simulink model "x4bus_model"  (R2024b)
settings: Solver=VariableStepAuto  StartTime=0.0  StopTime=4  RelTol=1e-3
InitFcn:
  |         %主电路参数
  | Vin = 800;    Vtri = 400;
  | Vg = 220;     Po = 100e3*1; Qo=0;
  | Po2 = Po;    Qo2 = 0;
  | Vg1 = Vg;
  | fline = 50;   fsw = 10e3;
  | fsample = 20e3;
  | wn = 2*pi*fline;
  | L1 = 3.2e-3;  C = 50e-6;
  | L2 = 800e-6;
  | Rcf = 0.8;
  | %% GFM1
  |         %有功功率环路参数
  | Dp = 1.59e4;  %EN 50438 要求频率变化49~51Hz
  | J = 0.081;
  |         %无功功率环路参数
  | Dq = 3210;
  | K = 7.1;
  | 
  | Rv = 0.6;Lv = 3.2e-3;
  | Kp_Vreg = 0.4;
  | Ki_Vreg = 90;
  | Kp_Ireg = 11;
  | Ki_Ireg = 0;
  | 
  | Ts = 1e-6;
  | 
  | t1 = 5;
  | t2 = 100;
  | 
  | %% GFM2
  |         %有功功率环路参数
  | Dp2 = 1.59e4;  %EN 50438 要求频率变化49~51Hz
  | J2 = 0.081;
  |         %无功功率环路参数
  | Dq2 = 3210;
  | K2 = 7.1;
  | 
  | Rv2 = 0.46;Lv2 = 0.8e-3;
  | Kp_Vreg2 = 0.3;   % 0.25
  | Ki_Vreg2 = 85;    % 80
  | Kp_Ireg2 = 11;
  | Ki_Ireg2 = 0;
undefined symbols (not defined in the file or in its folder): DiscIntNeverNeededParam, t_C, t_R
libraries: spsThreePhaseSeriesRLCBranchLib x13, spsCurrentMeasurementLib x12, spsControlledVoltageSourceLib x9, slpidlib x8, spsGroundLib x7, spsabctodq0Lib x6, spsVoltageMeasurementLib x6, spsThreePhaseBreakerLib x4, spsdq0toabcLib x3, spsFirstOrderFilterLib x2, sps_lib x1
(part 1 of 2)
settings Model: Creator=ZhenWei  LastModifiedBy=ZhenWei
settings DataIOCC: ReturnWorkspaceOutputs=off

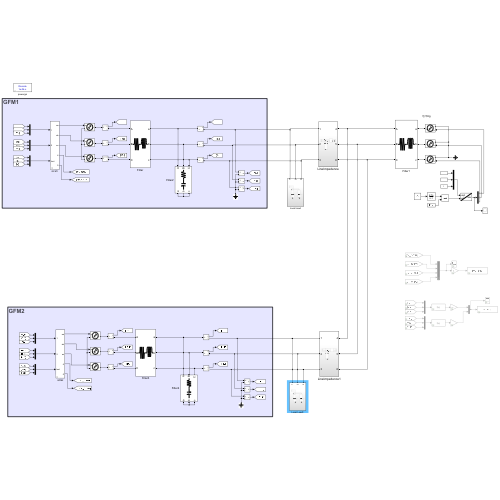
[thumbnail: Simulink's stored preview of the top-level diagram]
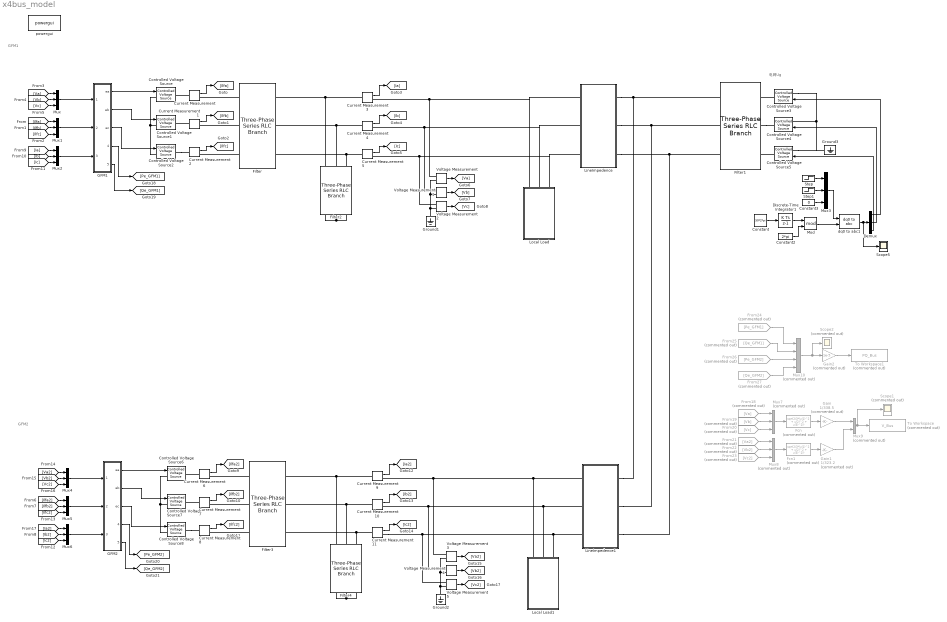
== system x4bus_model ==
  note: GFM1
  note: 电网Ug
  note: GFM2
  Constant : Constant  Value=50*2*pi
  Constant2 : Constant  Value=2*pi
  Constant3 : Constant  Value=0
  Controlled Voltage Source{,1..8} (9 alike) : spsControlledVoltageSourceLib/Controlled Voltage Source  Initialize=on  Source_Type=AC  Amplitude=0  Phase=0  Frequency=0  Measurements=None
  Current Measurement{,1..11} (12 alike) : spsCurrentMeasurementLib/Current Measurement  PhasorSimulation=off  OutputType=Complex  PSBequivalent=0
  Demux : Demux  Outputs=3
  Discrete-Time Integrator1 : DiscreteIntegrator  SampleTime=-1  ICPrevOutput=DiscIntNeverNeededParam  ICPrevScaledInput=DiscIntNeverNeededParam
  Fcn : Fcn  Commented=on  Expr=sqrt(2/3*(u(1)^2 + u(2)^2 + u(3)^2))
  Fcn1 : Fcn  Commented=on  Expr=sqrt(2/3*(u(1)^2 + u(2)^2 + u(3)^2))
  Filter : spsThreePhaseSeriesRLCBranchLib/Three-Phase Series RLC Branch  LConnTagsString=A|B|C  RConnTagsString=A|B|C  BranchType=RL  Resistance=0.05  Inductance=L1  Capacitance=1e-6  Measurements=None
  Filter1 : spsThreePhaseSeriesRLCBranchLib/Three-Phase Series RLC Branch  LConnTagsString=A|B|C  RConnTagsString=A|B|C  BranchType=RL  Resistance=0.01452  Inductance=0.462e-3  Capacitance=1e-6  Measurements=None
  Filter2 : spsThreePhaseSeriesRLCBranchLib/Three-Phase Series RLC Branch  LConnTagsString=A|B|C  RConnTagsString=A|B|C  BranchType=RC  Resistance=Rcf  Inductance=L2  Capacitance=C  Measurements=None
  Filter3 : spsThreePhaseSeriesRLCBranchLib/Three-Phase Series RLC Branch  LConnTagsString=A|B|C  RConnTagsString=A|B|C  BranchType=RL  Resistance=0.05  Inductance=L1  Capacitance=1e-6  Measurements=None
  Filter4 : spsThreePhaseSeriesRLCBranchLib/Three-Phase Series RLC Branch  LConnTagsString=A|B|C  RConnTagsString=A|B|C  BranchType=RC  Resistance=Rcf  Inductance=L2  Capacitance=C  Measurements=None
  From18 : From  Commented=on  GotoTag=Va
  From19 : From  Commented=on  GotoTag=Vb
  From20 : From  Commented=on  GotoTag=Vc
  From21 : From  Commented=on  GotoTag=Va2
  From22 : From  Commented=on  GotoTag=Vb2
  From23 : From  Commented=on  GotoTag=Vc2
  From24 : From  Commented=on  GotoTag=Pe_GFM1
  From25 : From  Commented=on  GotoTag=Qe_GFM1
  From26 : From  Commented=on  GotoTag=Pe_GFM2
  From27 : From  Commented=on  GotoTag=Qe_GFM2
  GFM1 : Subsystem  mask{J=J, Dp=Dp, Dq=Dq, K=K, Kp_Vreg=Kp_Vreg, Ki_Vreg=Ki_Vreg, Kp_Ireg=Kp_Ireg, Ki_Ireg=Ki_Ireg, Lv=Lv, Rv=Rv, Po=Po, Qo=Qo}
      mask prompts: J "惯性系数J"; Dp "有功阻尼Dp"; Dq "无功阻尼Dq"; K "下垂系数K"; Kp_Vreg "电压环kp"; Ki_Vreg "电压环ki"; Kp_Ireg "电流环kp"; Ki_Ireg "电流环ki"; Lv "虚拟电感Lv"; Rv "虚拟电阻Rv"; Po "有功功率Po"; Qo "无功功率Qo"
      mask DialogControl ParameterGroupVar Prompt: 参数
  GFM2 : Subsystem  mask{J=J2, Dp=Dp2, Dq=Dq2, K=K2, Kp_Vreg=Kp_Vreg2, Ki_Vreg=Ki_Vreg2, Kp_Ireg=Kp_Ireg2, Ki_Ireg=Ki_Ireg2, Lv=Lv2, Rv=Rv2, Po=Po2, Qo=Qo2}
      mask prompts: J "惯性系数J"; Dp "有功阻尼Dp"; Dq "无功阻尼Dq"; K "下垂系数K"; Kp_Vreg "电压环kp"; Ki_Vreg "电压环ki"; Kp_Ireg "电流环kp"; Ki_Ireg "电流环ki"; Lv "虚拟电感Lv"; Rv "虚拟电阻Rv"; Po "有功功率Po"; Qo "无功功率Qo"
      mask DialogControl ParameterGroupVar Prompt: 参数
  Gain : Gain  Commented=on  Gain=1/338.5
  Gain1 : Gain  Commented=on  Gain=1/323.2
  Gain2 : Gain  Commented=on  Gain=1e-5
  Ground1 : spsGroundLib/Ground  LConnTagsString=a
  Ground2 : spsGroundLib/Ground  LConnTagsString=a
  Ground3 : spsGroundLib/Ground  LConnTagsString=a
  LineImpedence : Subsystem
  LineImpedence1 : Subsystem
  Local Load : Subsystem
  Local Load1 : Subsystem
  Mod : Math  Operator=mod
  Mux{,1..6} (7 alike) : Mux  Inputs=3
  Mux10 : Mux  Commented=on
  Mux7 : Mux  Commented=on  Inputs=3
  Mux8 : Mux  Commented=on  Inputs=3
  Mux9 : Mux  Commented=on  Inputs=2
  Scope1 : Scope  Commented=on
  Scope2 : Scope  Commented=on
  Scope5 : Scope
  Step : Step  Time=10  Before=311  After=311+20  SampleTime=0
  Step1 : Step  Time=10  After=30  SampleTime=0
  To Workspace : ToWorkspace  Commented=on  VariableName=V_Bus  SaveFormat=Timeseries  SampleTime=-1
  To Workspace1 : ToWorkspace  Commented=on  VariableName=PQ_Bus  SaveFormat=Timeseries  SampleTime=-1
  Voltage Measurement{,1..5} (6 alike) : spsVoltageMeasurementLib/Voltage Measurement  PhasorSimulation=off  OutputType=Complex  PSBequivalent=0
  dq0 to abc1 : spsdq0toabcLib/dq0 to abc  Alignment=90 degrees behind phase A axis
  powergui : sps_lib/powergui  Priority=1  SimulationMode=Discrete  SampleTime=1e-6  frequency=60  Iterations=50  frequencyindice=0  Pbase=100e6  ErrMax=1e-4  UnitsV=kV  UnitsW=MW  buscounter=0  FunctionMessages=off  echomessages=off  EnableUseOfTLC=off  CurrentSourceSwitches=off  DisableSnubberDevices=off  DisableRonSwitches=off  DisableVfSwitches=off  DisplayEquations=off  AutomaticDiscreteSolvers=off  SolverType=Tustin/Backward Euler (TBE)  Interpol=off  ExternalGateDelay=off  methode=off  Ts=100  x0status=blocks  SPID=on  SwTol=0  HookPort=off  NonlinearTolerance=1e-4  nMaxIteration=100  ContinueOnMaxIteration=off  RestoreLinks=warning  ResistiveCurrentMeasurement=off  Frange=[0:2:500]  Ylog=off  Xlog=on  ShowGrid=off  save=off  variable=ZData  structure=0  ZoomFFT=off  StartTime=0.0  cycles=1  DisplayStyle=1  fundamental=60  FreqAxis=off  MaxFrequency=1000  frequencyindicesteady=1  RmsSteady=1  display=off
  wires:
  Current Measurement/1 -> [Ilfa]
  Current Measurement1/1 -> [Ilfb]
  Current Measurement2/1 -> [Ilfc]
  Current Measurement3/1 -> [Ia]
  Current Measurement4/1 -> [Ib]
  Current Measurement5/1 -> [Ic]
  Voltage Measurement/1 -> [Va]
  Voltage Measurement1/1 -> [Vb]
  Voltage Measurement2/1 -> [Vc]
  GFM1/1(ea) -> Controlled Voltage Source/1
  GFM1/2(eb) -> Controlled Voltage Source1/1
  GFM1/3(ec) -> Controlled Voltage Source2/1
  [Va] -> Mux/1
  [Vb] -> Mux/2
  [Vc] -> Mux/3
  [Ilfa] -> Mux1/1
  [Ilfb] -> Mux1/2
  [Ilfc] -> Mux1/3
  [Ic] -> Mux2/3
  [Ib] -> Mux2/2
  [Ia] -> Mux2/1
  Mux/1 -> GFM1/1(Inport)
  Mux1/1 -> GFM1/2(Inport1)
  Mux2/1 -> GFM1/3(Iout)
  Constant/1 -> Discrete-Time Integrator1/1
  Discrete-Time Integrator1/1 -> Mod/1
  Constant2/1 -> Mod/2
  Mod/1 -> dq0 to abc1/2
  Step/1 -> Mux3/1
  Constant3/1 -> Mux3/3
  Mux3/1 -> dq0 to abc1/1
  dq0 to abc1/1 -> Scope5/1, Demux/1
  Demux/1 -> Controlled Voltage Source3/1
  Demux/2 -> Controlled Voltage Source4/1
  Demux/3 -> Controlled Voltage Source5/1
  Step1/1 -> Mux3/2
  Mux6/1 -> GFM2/3(Iout)
  Mux5/1 -> GFM2/2(Inport1)
  Mux4/1 -> GFM2/1(Inport)
  [Ia2] -> Mux6/1
  [Ib2] -> Mux6/2
  [Ic2] -> Mux6/3
  [Ilfc2] -> Mux5/3
  [Ilfb2] -> Mux5/2
  [Ilfa2] -> Mux5/1
  [Vc2] -> Mux4/3
  [Vb2] -> Mux4/2
  [Va2] -> Mux4/1
  GFM2/3(ec) -> Controlled Voltage Source8/1
  GFM2/2(eb) -> Controlled Voltage Source7/1
  GFM2/1(ea) -> Controlled Voltage Source6/1
  Voltage Measurement5/1 -> [Vc2]
  Voltage Measurement4/1 -> [Vb2]
  Voltage Measurement3/1 -> [Va2]
  Current Measurement11/1 -> [Ic2]
  Current Measurement10/1 -> [Ib2]
  Current Measurement9/1 -> [Ia2]
  Current Measurement8/1 -> [Ilfc2]
  Current Measurement7/1 -> [Ilfb2]
  Current Measurement6/1 -> [Ilfa2]
  Mux7/1 -> Fcn/1
  From18/1 -> Mux7/1
  From19/1 -> Mux7/2
  From20/1 -> Mux7/3
  Fcn/1 -> Gain/1
  From23/1 -> Mux8/3
  From22/1 -> Mux8/2
  From21/1 -> Mux8/1
  Mux8/1 -> Fcn1/1
  Fcn1/1 -> Gain1/1
  Gain/1 -> Mux9/1
  Gain1/1 -> Mux9/2
  Mux9/1 -> Scope1/1, To Workspace/1
  GFM1/4(Out1) -> [Pe_GFM1]
  GFM1/5(Out2) -> [Qe_GFM1]
  GFM2/4(Out1) -> [Pe_GFM2]
  GFM2/5(Out2) -> [Qe_GFM2]
  Mux10/1 -> Scope2/1, Gain2/1
  From24/1 -> Mux10/1
  From25/1 -> Mux10/2
  From26/1 -> Mux10/3
  From27/1 -> Mux10/4
  Gain2/1 -> To Workspace1/1
  connections:
  Controlled Voltage Source/LConn1 -- Controlled Voltage Source2/LConn1 -- Controlled Voltage Source1/LConn1
  Current Measurement/LConn1 -- Controlled Voltage Source/RConn1
  Current Measurement1/LConn1 -- Controlled Voltage Source1/RConn1
  Controlled Voltage Source2/RConn1 -- Current Measurement2/LConn1
  Filter2/LConn2 -- Current Measurement4/LConn1 -- Filter/RConn2
  Filter2/LConn1 -- Current Measurement3/LConn1 -- Filter/RConn1
  Filter2/RConn1 -- Filter2/RConn2 -- Filter2/RConn3
  Filter2/LConn3 -- Current Measurement5/LConn1 -- Filter/RConn3
  Filter/LConn2 -- Current Measurement1/RConn1
  Filter/LConn1 -- Current Measurement/RConn1
  Filter/LConn3 -- Current Measurement2/RConn1
  Filter1/RConn2 -- Controlled Voltage Source4/RConn1
  Controlled Voltage Source3/RConn1 -- Filter1/RConn1
  Controlled Voltage Source5/RConn1 -- Filter1/RConn3
  Voltage Measurement/LConn1 -- LineImpedence/LConn1 -- Local Load/LConn1 -- Current Measurement3/RConn1
  Voltage Measurement1/LConn1 -- LineImpedence/LConn2 -- Local Load/LConn2 -- Current Measurement4/RConn1
  Voltage Measurement/LConn2 -- Voltage Measurement1/LConn2 -- Ground1/LConn1 -- Voltage Measurement2/LConn2
  Controlled Voltage Source3/LConn1 -- Controlled Voltage Source5/LConn1 -- Ground3/LConn1 -- Controlled Voltage Source4/LConn1
  Voltage Measurement2/LConn1 -- LineImpedence/LConn3 -- Local Load/LConn3 -- Current Measurement5/RConn1
  Controlled Voltage Source6/LConn1 -- Controlled Voltage Source7/LConn1 -- Controlled Voltage Source8/LConn1
  Filter4/LConn2 -- Current Measurement10/LConn1 -- Filter3/RConn2
  Filter4/LConn1 -- Current Measurement9/LConn1 -- Filter3/RConn1
  Filter4/RConn1 -- Filter4/RConn3 -- Filter4/RConn2
  Filter4/LConn3 -- Filter3/RConn3 -- Current Measurement11/LConn1
  Voltage Measurement3/LConn2 -- Voltage Measurement5/LConn2 -- Ground2/LConn1 -- Voltage Measurement4/LConn2
  Filter3/LConn3 -- Current Measurement8/RConn1
  Filter3/LConn2 -- Current Measurement7/RConn1
  Filter3/LConn1 -- Current Measurement6/RConn1
  Current Measurement7/LConn1 -- Controlled Voltage Source7/RConn1
  Controlled Voltage Source8/RConn1 -- Current Measurement8/LConn1
  Current Measurement6/LConn1 -- Controlled Voltage Source6/RConn1
  LineImpedence/RConn1 -- LineImpedence1/RConn1 -- Filter1/LConn1
  LineImpedence/RConn2 -- LineImpedence1/RConn2 -- Filter1/LConn2
  LineImpedence/RConn3 -- LineImpedence1/RConn3 -- Filter1/LConn3
  LineImpedence1/LConn1 -- Current Measurement9/RConn1 -- Voltage Measurement3/LConn1 -- Local Load1/LConn1
  LineImpedence1/LConn2 -- Local Load1/LConn2 -- Voltage Measurement4/LConn1 -- Current Measurement10/RConn1
  Current Measurement11/RConn1 -- Voltage Measurement5/LConn1 -- Local Load1/LConn3 -- LineImpedence1/LConn3

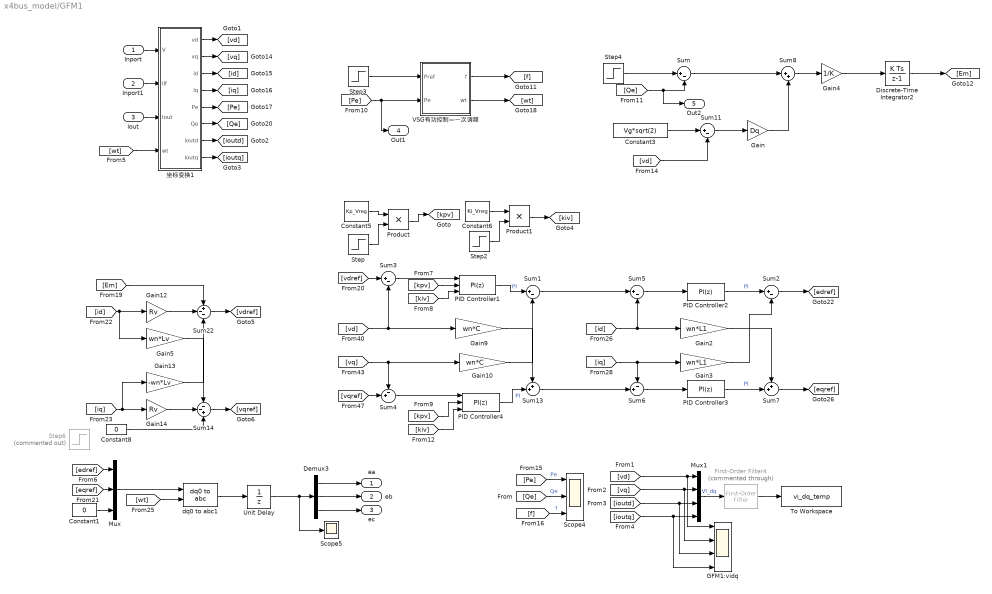
== system x4bus_model/GFM1 ==
  Inport : Inport
  Inport1 : Inport  Port=2
  Iout : Inport  Port=3
  Constant1 : Constant  Value=0
  Constant3 : Constant  Value=Vg*sqrt(2)
  Constant5 : Constant  Value=Kp_Vreg
  Constant6 : Constant  Value=Ki_Vreg
  Constant8 : Constant  Value=0
  Demux3 : Demux  Outputs=3
  Discrete-Time Integrator2 : DiscreteIntegrator  SampleTime=-1  ICPrevOutput=DiscIntNeverNeededParam  ICPrevScaledInput=DiscIntNeverNeededParam
  First-Order Filter4 : spsFirstOrderFilterLib/First-Order Filter  Commented=through  FilterType=Lowpass  Tc=5e-3  Ts=Ts  Initialize=off  Vac_Init=[0, 0, 1000]  Vdc_Init=0  PlotResponse=off  FreqRange="[0,  200,  1]"
  GFM1:vidq : Scope  NumInputPorts=4
  Gain : Gain  Gain=Dq
  Gain10 : Gain  Gain=wn*C
  Gain12 : Gain  Gain=Rv
  Gain13 : Gain  Gain=-wn*Lv
  Gain14 : Gain  Gain=Rv
  Gain2 : Gain  Gain=wn*L1
  Gain3 : Gain  Gain=wn*L1
  Gain4 : Gain  Gain=1/K
  Gain5 : Gain  Gain=wn*Lv
  Gain9 : Gain  Gain=wn*C
  Mux : Mux  Inputs=3
  Mux1 : Mux
  PID Controller1 : slpidlib/PID Controller  Controller=PI  Form=Parallel  TimeDomain=Discrete-time  UseExternalTs=off  SampleTime=-1  IntegratorMethod=Forward Euler  FilterMethod=Forward Euler  ControllerParametersSource=external  P=Kp_Vreg  I=Ki_Vreg  UseKiTs=off  D=0  UseExternalDerivativeSource=off  N=100  UseFilter=on  TunerSelectOption=Transfer Function Based (PID Tuner App)  InitialConditionSource=internal  InitialConditionForIntegrator=0  InitialConditionForFilter=0  DifferentiatorICPrevScaledInput=0  ExternalReset=none  TrackingMode=off  Kt=1  LimitOutput=off  SatLimitsSource=internal  UpperSaturationLimit=inf  LowerSaturationLimit=-inf  LinearizeAsGain=on  AntiWindupMode=none  Kb=1  LimitIntegrator=off  UpperIntegratorSaturationLimit=inf  LowerIntegratorSaturationLimit=-inf  POutMin=[]  POutMax=[]  IOutMin=[]  IOutMax=[]  DOutMin=[]  DOutMax=[]  NOutMin=[]  NOutMax=[]  SumOutMin=[]  SumOutMax=[]  SaturationOutMin=[]  SaturationOutMax=[]  PParamMin=[]  PParamMax=[]  IParamMin=[]  IParamMax=[]  DParamMin=[]  DParamMax=[]  NParamMin=[]  NParamMax=[]  KbParamMin=[]  KbParamMax=[]  KtParamMin=[]  KtParamMax=[]  KbOutMin=[]  KbOutMax=[]  KtOutMin=[]  KtOutMax=[]  IntegratorOutMin=[]  IntegratorOutMax=[]  FilterOutMin=[]  FilterOutMax=[]  SumI1OutMin=[]  SumI1OutMax=[]  SumI2OutMin=[]  SumI2OutMax=[]  SumI3OutMin=[]  SumI3OutMax=[]  SumI4OutMin=[]  SumI4OutMax=[]  SumDOutMin=[]  SumDOutMax=[]  DifferentiatorOutMin=[]  DifferentiatorOutMax=[]  FilterDiffOutCoefMin=[]  FilterDiffOutCoefMax=[]  ReciprocalOutMin=[]  ReciprocalOutMax=[]  SumDenOutMin=[]  SumDenOutMax=[]  SumNumOutMin=[]  SumNumOutMax=[]  DivideOutMin=[]  DivideOutMax=[]  UdiffTsProdOutMin=[]  UdiffTsProdOutMax=[]  NTsProdOutMin=[]  NTsProdOutMax=[]  UintegralTsProdOutMin=[]  UintegralTsProdOutMax=[]  UngainTsProdOutMin=[]  UngainTsProdOutMax=[]  ClampingZeroOutDataTypeStr=Inherit: Inherit via back propagation  ClampingZeroOutMin=[]  ClampingZeroOutMax=[]  FilterDenConstantOutDataTypeStr=Inherit: Inherit via back propagation  FilterDenConstantOutMin=[]  FilterDenConstantOutMax=[]  PCopyOutDataTypeStr=Inherit: Inherit via back propagation  PCopyOutMin=[]  PCopyOutMax=[]  NCopyOutDataTypeStr=Inherit: Inherit via back propagation  NCopyOutMin=[]  NCopyOutMax=[]  IntegratorContinuousStateAttributes=''  IntegratorStateMustResolveToSignalObject=off  IntegratorRTWStateStorageClass=Auto  FilterContinuousStateAttributes=''  FilterStateMustResolveToSignalObject=off  FilterRTWStateStorageClass=Auto  ParallelPVariant=ExternalParameters  IdealPVariant=Disabled  IVariant=ExternalParameters  DVariant=Disabled  IntegratorVariant=Discrete  SatVariant=Disabled  AWVariant=Passthrough  PCopyVariant=Disabled  TRVariant=Disabled  FdbkBlocksVariant=Forward  IdealPFdbkVariant=Disabled  SatFdbkVariant=Disabled  DerivativeFilterVariant=Disabled  NVariant=Disabled  NCopyVariant=Disabled_SignalSpec  FilterICVariant=Disabled  IntegratorICVariant=InternalICs  ExternalResetVariant=Disabled  TRSumVariant=Passthrough  SumFdbkVariant=Disabled  SumVariant=Sum_PI  TsampFilterVariant=InternalTs  TsampNgainVariant=Passthrough  TsampIntegralVariant=Disabled_SignalSpec  ExternalSaturationOutDataTypeStr=Inherit: Same as second input  DerivativeSourceVariant=Disabled  PreIntVariant=InternalPreInt
  PID Controller2 : slpidlib/PID Controller  Controller=PI  Form=Parallel  TimeDomain=Discrete-time  UseExternalTs=off  SampleTime=-1  IntegratorMethod=Forward Euler  FilterMethod=Forward Euler  ControllerParametersSource=internal  P=Kp_Ireg  I=Ki_Ireg  UseKiTs=off  D=0  UseExternalDerivativeSource=off  N=100  UseFilter=on  TunerSelectOption=Transfer Function Based (PID Tuner App)  InitialConditionSource=internal  InitialConditionForIntegrator=0  InitialConditionForFilter=0  DifferentiatorICPrevScaledInput=0  ExternalReset=none  TrackingMode=off  Kt=1  LimitOutput=off  SatLimitsSource=internal  UpperSaturationLimit=inf  LowerSaturationLimit=-inf  LinearizeAsGain=on  AntiWindupMode=none  Kb=1  LimitIntegrator=off  UpperIntegratorSaturationLimit=inf  LowerIntegratorSaturationLimit=-inf  POutMin=[]  POutMax=[]  IOutMin=[]  IOutMax=[]  DOutMin=[]  DOutMax=[]  NOutMin=[]  NOutMax=[]  SumOutMin=[]  SumOutMax=[]  SaturationOutMin=[]  SaturationOutMax=[]  PParamMin=[]  PParamMax=[]  IParamMin=[]  IParamMax=[]  DParamMin=[]  DParamMax=[]  NParamMin=[]  NParamMax=[]  KbParamMin=[]  KbParamMax=[]  KtParamMin=[]  KtParamMax=[]  KbOutMin=[]  KbOutMax=[]  KtOutMin=[]  KtOutMax=[]  IntegratorOutMin=[]  IntegratorOutMax=[]  FilterOutMin=[]  FilterOutMax=[]  SumI1OutMin=[]  SumI1OutMax=[]  SumI2OutMin=[]  SumI2OutMax=[]  SumI3OutMin=[]  SumI3OutMax=[]  SumI4OutMin=[]  SumI4OutMax=[]  SumDOutMin=[]  SumDOutMax=[]  DifferentiatorOutMin=[]  DifferentiatorOutMax=[]  FilterDiffOutCoefMin=[]  FilterDiffOutCoefMax=[]  ReciprocalOutMin=[]  ReciprocalOutMax=[]  SumDenOutMin=[]  SumDenOutMax=[]  SumNumOutMin=[]  SumNumOutMax=[]  DivideOutMin=[]  DivideOutMax=[]  UdiffTsProdOutMin=[]  UdiffTsProdOutMax=[]  NTsProdOutMin=[]  NTsProdOutMax=[]  UintegralTsProdOutMin=[]  UintegralTsProdOutMax=[]  UngainTsProdOutMin=[]  UngainTsProdOutMax=[]  ClampingZeroOutDataTypeStr=Inherit: Inherit via back propagation  ClampingZeroOutMin=[]  ClampingZeroOutMax=[]  FilterDenConstantOutDataTypeStr=Inherit: Inherit via back propagation  FilterDenConstantOutMin=[]  FilterDenConstantOutMax=[]  PCopyOutDataTypeStr=Inherit: Inherit via back propagation  PCopyOutMin=[]  PCopyOutMax=[]  NCopyOutDataTypeStr=Inherit: Inherit via back propagation  NCopyOutMin=[]  NCopyOutMax=[]  IntegratorContinuousStateAttributes=''  IntegratorStateMustResolveToSignalObject=off  IntegratorRTWStateStorageClass=Auto  FilterContinuousStateAttributes=''  FilterStateMustResolveToSignalObject=off  FilterRTWStateStorageClass=Auto  ParallelPVariant=InternalParameters  IdealPVariant=Disabled  IVariant=InternalParameters  DVariant=Disabled  IntegratorVariant=Discrete  SatVariant=Disabled  AWVariant=Passthrough  PCopyVariant=Disabled  TRVariant=Disabled  FdbkBlocksVariant=Forward  IdealPFdbkVariant=Disabled  SatFdbkVariant=Disabled  DerivativeFilterVariant=Disabled  NVariant=Disabled  NCopyVariant=Disabled_SignalSpec  FilterICVariant=Disabled  IntegratorICVariant=InternalICs  ExternalResetVariant=Disabled  TRSumVariant=Passthrough  SumFdbkVariant=Disabled  SumVariant=Sum_PI  TsampFilterVariant=InternalTs  TsampNgainVariant=Passthrough  TsampIntegralVariant=Disabled_SignalSpec  ExternalSaturationOutDataTypeStr=Inherit: Same as second input  DerivativeSourceVariant=Disabled  PreIntVariant=InternalPreInt
  PID Controller3 : slpidlib/PID Controller  Controller=PI  Form=Parallel  TimeDomain=Discrete-time  UseExternalTs=off  SampleTime=-1  IntegratorMethod=Forward Euler  FilterMethod=Forward Euler  ControllerParametersSource=internal  P=Kp_Ireg  I=Ki_Ireg  UseKiTs=off  D=0  UseExternalDerivativeSource=off  N=100  UseFilter=on  TunerSelectOption=Transfer Function Based (PID Tuner App)  InitialConditionSource=internal  InitialConditionForIntegrator=0  InitialConditionForFilter=0  DifferentiatorICPrevScaledInput=0  ExternalReset=none  TrackingMode=off  Kt=1  LimitOutput=off  SatLimitsSource=internal  UpperSaturationLimit=inf  LowerSaturationLimit=-inf  LinearizeAsGain=on  AntiWindupMode=none  Kb=1  LimitIntegrator=off  UpperIntegratorSaturationLimit=inf  LowerIntegratorSaturationLimit=-inf  POutMin=[]  POutMax=[]  IOutMin=[]  IOutMax=[]  DOutMin=[]  DOutMax=[]  NOutMin=[]  NOutMax=[]  SumOutMin=[]  SumOutMax=[]  SaturationOutMin=[]  SaturationOutMax=[]  PParamMin=[]  PParamMax=[]  IParamMin=[]  IParamMax=[]  DParamMin=[]  DParamMax=[]  NParamMin=[]  NParamMax=[]  KbParamMin=[]  KbParamMax=[]  KtParamMin=[]  KtParamMax=[]  KbOutMin=[]  KbOutMax=[]  KtOutMin=[]  KtOutMax=[]  IntegratorOutMin=[]  IntegratorOutMax=[]  FilterOutMin=[]  FilterOutMax=[]  SumI1OutMin=[]  SumI1OutMax=[]  SumI2OutMin=[]  SumI2OutMax=[]  SumI3OutMin=[]  SumI3OutMax=[]  SumI4OutMin=[]  SumI4OutMax=[]  SumDOutMin=[]  SumDOutMax=[]  DifferentiatorOutMin=[]  DifferentiatorOutMax=[]  FilterDiffOutCoefMin=[]  FilterDiffOutCoefMax=[]  ReciprocalOutMin=[]  ReciprocalOutMax=[]  SumDenOutMin=[]  SumDenOutMax=[]  SumNumOutMin=[]  SumNumOutMax=[]  DivideOutMin=[]  DivideOutMax=[]  UdiffTsProdOutMin=[]  UdiffTsProdOutMax=[]  NTsProdOutMin=[]  NTsProdOutMax=[]  UintegralTsProdOutMin=[]  UintegralTsProdOutMax=[]  UngainTsProdOutMin=[]  UngainTsProdOutMax=[]  ClampingZeroOutDataTypeStr=Inherit: Inherit via back propagation  ClampingZeroOutMin=[]  ClampingZeroOutMax=[]  FilterDenConstantOutDataTypeStr=Inherit: Inherit via back propagation  FilterDenConstantOutMin=[]  FilterDenConstantOutMax=[]  PCopyOutDataTypeStr=Inherit: Inherit via back propagation  PCopyOutMin=[]  PCopyOutMax=[]  NCopyOutDataTypeStr=Inherit: Inherit via back propagation  NCopyOutMin=[]  NCopyOutMax=[]  IntegratorContinuousStateAttributes=''  IntegratorStateMustResolveToSignalObject=off  IntegratorRTWStateStorageClass=Auto  FilterContinuousStateAttributes=''  FilterStateMustResolveToSignalObject=off  FilterRTWStateStorageClass=Auto  ParallelPVariant=InternalParameters  IdealPVariant=Disabled  IVariant=InternalParameters  DVariant=Disabled  IntegratorVariant=Discrete  SatVariant=Disabled  AWVariant=Passthrough  PCopyVariant=Disabled  TRVariant=Disabled  FdbkBlocksVariant=Forward  IdealPFdbkVariant=Disabled  SatFdbkVariant=Disabled  DerivativeFilterVariant=Disabled  NVariant=Disabled  NCopyVariant=Disabled_SignalSpec  FilterICVariant=Disabled  IntegratorICVariant=InternalICs  ExternalResetVariant=Disabled  TRSumVariant=Passthrough  SumFdbkVariant=Disabled  SumVariant=Sum_PI  TsampFilterVariant=InternalTs  TsampNgainVariant=Passthrough  TsampIntegralVariant=Disabled_SignalSpec  ExternalSaturationOutDataTypeStr=Inherit: Same as second input  DerivativeSourceVariant=Disabled  PreIntVariant=InternalPreInt
  PID Controller4 : slpidlib/PID Controller  Controller=PI  Form=Parallel  TimeDomain=Discrete-time  UseExternalTs=off  SampleTime=-1  IntegratorMethod=Forward Euler  FilterMethod=Forward Euler  ControllerParametersSource=external  P=Kp_Vreg  I=Ki_Vreg  UseKiTs=off  D=0  UseExternalDerivativeSource=off  N=100  UseFilter=on  TunerSelectOption=Transfer Function Based (PID Tuner App)  InitialConditionSource=internal  InitialConditionForIntegrator=0  InitialConditionForFilter=0  DifferentiatorICPrevScaledInput=0  ExternalReset=none  TrackingMode=off  Kt=1  LimitOutput=off  SatLimitsSource=internal  UpperSaturationLimit=inf  LowerSaturationLimit=-inf  LinearizeAsGain=on  AntiWindupMode=none  Kb=1  LimitIntegrator=off  UpperIntegratorSaturationLimit=inf  LowerIntegratorSaturationLimit=-inf  POutMin=[]  POutMax=[]  IOutMin=[]  IOutMax=[]  DOutMin=[]  DOutMax=[]  NOutMin=[]  NOutMax=[]  SumOutMin=[]  SumOutMax=[]  SaturationOutMin=[]  SaturationOutMax=[]  PParamMin=[]  PParamMax=[]  IParamMin=[]  IParamMax=[]  DParamMin=[]  DParamMax=[]  NParamMin=[]  NParamMax=[]  KbParamMin=[]  KbParamMax=[]  KtParamMin=[]  KtParamMax=[]  KbOutMin=[]  KbOutMax=[]  KtOutMin=[]  KtOutMax=[]  IntegratorOutMin=[]  IntegratorOutMax=[]  FilterOutMin=[]  FilterOutMax=[]  SumI1OutMin=[]  SumI1OutMax=[]  SumI2OutMin=[]  SumI2OutMax=[]  SumI3OutMin=[]  SumI3OutMax=[]  SumI4OutMin=[]  SumI4OutMax=[]  SumDOutMin=[]  SumDOutMax=[]  DifferentiatorOutMin=[]  DifferentiatorOutMax=[]  FilterDiffOutCoefMin=[]  FilterDiffOutCoefMax=[]  ReciprocalOutMin=[]  ReciprocalOutMax=[]  SumDenOutMin=[]  SumDenOutMax=[]  SumNumOutMin=[]  SumNumOutMax=[]  DivideOutMin=[]  DivideOutMax=[]  UdiffTsProdOutMin=[]  UdiffTsProdOutMax=[]  NTsProdOutMin=[]  NTsProdOutMax=[]  UintegralTsProdOutMin=[]  UintegralTsProdOutMax=[]  UngainTsProdOutMin=[]  UngainTsProdOutMax=[]  ClampingZeroOutDataTypeStr=Inherit: Inherit via back propagation  ClampingZeroOutMin=[]  ClampingZeroOutMax=[]  FilterDenConstantOutDataTypeStr=Inherit: Inherit via back propagation  FilterDenConstantOutMin=[]  FilterDenConstantOutMax=[]  PCopyOutDataTypeStr=Inherit: Inherit via back propagation  PCopyOutMin=[]  PCopyOutMax=[]  NCopyOutDataTypeStr=Inherit: Inherit via back propagation  NCopyOutMin=[]  NCopyOutMax=[]  IntegratorContinuousStateAttributes=''  IntegratorStateMustResolveToSignalObject=off  IntegratorRTWStateStorageClass=Auto  FilterContinuousStateAttributes=''  FilterStateMustResolveToSignalObject=off  FilterRTWStateStorageClass=Auto  ParallelPVariant=ExternalParameters  IdealPVariant=Disabled  IVariant=ExternalParameters  DVariant=Disabled  IntegratorVariant=Discrete  SatVariant=Disabled  AWVariant=Passthrough  PCopyVariant=Disabled  TRVariant=Disabled  FdbkBlocksVariant=Forward  IdealPFdbkVariant=Disabled  SatFdbkVariant=Disabled  DerivativeFilterVariant=Disabled  NVariant=Disabled  NCopyVariant=Disabled_SignalSpec  FilterICVariant=Disabled  IntegratorICVariant=InternalICs  ExternalResetVariant=Disabled  TRSumVariant=Passthrough  SumFdbkVariant=Disabled  SumVariant=Sum_PI  TsampFilterVariant=InternalTs  TsampNgainVariant=Passthrough  TsampIntegralVariant=Disabled_SignalSpec  ExternalSaturationOutDataTypeStr=Inherit: Same as second input  DerivativeSourceVariant=Disabled  PreIntVariant=InternalPreInt
  Product : Product
  Product1 : Product
  Scope4 : Scope  NumInputPorts=3
  Scope5 : Scope
  Step : Step  Time=t1  Before=1  After=0.85  SampleTime=0
  Step2 : Step  Time=t1  Before=1  After=0.9  SampleTime=0
  Step3 : Step  Time=t1  Before=Po  After=-1*Po  SampleTime=0
  Step4 : Step  Time=t1  Before=Qo  After=1*Po  SampleTime=0
  Step6 : Step  Commented=on  Time=10  After=20  SampleTime=0
  Sum{,1..3,5,11} (6 alike) : Sum  Inputs=|+-
  Sum13 : Sum  Inputs=++|
  Sum14 : Sum  Inputs=--+
  Sum22 : Sum  Inputs=+--
  Sum4 : Sum  Inputs=-+|
  Sum6 : Sum  Inputs=-+|
  Sum7 : Sum  Inputs=++|
  Sum8 : Sum  Inputs=|++
  To Workspace : ToWorkspace  VariableName=vi_dq_temp  SaveFormat=Timeseries  SampleTime=-1
  Unit Delay : UnitDelay  SampleTime=-1  HasFrameUpgradeWarning=on
  VSG有功控制—一次调频 : Subsystem
  dq0 to abc1 : spsdq0toabcLib/dq0 to abc  Alignment=90 degrees behind phase A axis
  坐标变换1 : Subsystem
  ea : Outport
  eb : Outport  Port=2
  ec : Outport  Port=3
  Out1 : Outport  Port=4
  Out2 : Outport  Port=5
  wires:
  [Pe] -> Scope4/1  "Pe"
  [f] -> Scope4/3  "f"
  [Qe] -> Scope4/2  "Qe"
  [vq] -> GFM1:vidq/2, Mux1/2
  [ioutd] -> GFM1:vidq/3, Mux1/3
  [vd] -> GFM1:vidq/1, Mux1/1
  [ioutq] -> GFM1:vidq/4, Mux1/4
  Mux1/1 -> First-Order Filter4/1  "VI_dq"
  First-Order Filter4/1 -> To Workspace/1
  Inport1/1 -> 坐标变换1/2(Ilf)
  [wt] -> 坐标变换1/4(wt)
  坐标变换1/1(vd) -> [vd]
  坐标变换1/2(vq) -> [vq]
  坐标变换1/3(id) -> [id]
  坐标变换1/4(iq) -> [iq]
  坐标变换1/5(Pe) -> [Pe]
  坐标变换1/6(Qe) -> [Qe]
  [wt] -> dq0 to abc1/2
  [edref] -> Mux/1
  [eqref] -> Mux/2
  Mux/1 -> dq0 to abc1/1
  Constant1/1 -> Mux/3
  dq0 to abc1/1 -> Unit Delay/1
  Demux3/1 -> ea/1
  Demux3/2 -> eb/1
  Demux3/3 -> ec/1
  Unit Delay/1 -> Scope5/1, Demux3/1
  Inport/1 -> 坐标变换1/1(V)
  坐标变换1/8(ioutq) -> [ioutq]
  坐标变换1/7(ioutd) -> [ioutd]
  Iout/1 -> 坐标变换1/3(Iout)
  Gain14/1 -> Sum14/2
  Gain12/1 -> Sum22/2
  [Em] -> Sum22/1
  Constant8/1 -> Sum14/3
  Sum14/1 -> [vqref]
  [id] -> Gain5/1, Gain12/1
  Gain13/1 -> Sum22/3
  Gain5/1 -> Sum14/1
  Sum22/1 -> [vdref]
  [iq] -> Gain13/1, Gain14/1
  [Pe] -> Out1/1, VSG有功控制—一次调频/2(Pe)
  VSG有功控制—一次调频/2(wt) -> [wt]
  VSG有功控制—一次调频/1(f) -> [f]
  [vd] -> Sum11/2
  Step4/1 -> Sum/1
  [Qe] -> Out2/1, Sum/2
  Sum/1 -> Sum8/1
  Gain/1 -> Sum8/2
  Gain4/1 -> Discrete-Time Integrator2/1
  Sum11/1 -> Gain/1
  Step3/1 -> VSG有功控制—一次调频/1(Pref)
  Sum8/1 -> Gain4/1
  Constant3/1 -> Sum11/1
  Discrete-Time Integrator2/1 -> [Em]
  Product1/1 -> [kiv]
  [kiv] -> PID Controller1/3
  Sum13/1 -> Sum6/2
  [kpv] -> PID Controller4/2
  Sum1/1 -> Sum5/1
  Step/1 -> Product/2
  Step2/1 -> Product1/2
  Sum5/1 -> PID Controller2/1
  Sum2/1 -> [edref]
  Sum4/1 -> PID Controller4/1
  Sum6/1 -> PID Controller3/1
  [kiv] -> PID Controller4/3
  Gain3/1 -> Sum2/2
  PID Controller3/1 -> Sum7/2  "PI"
  Sum3/1 -> PID Controller1/1
  [vq] -> Gain10/1, Sum4/1
  [iq] -> Sum6/1, Gain3/1
  Gain9/1 -> Sum13/1
  PID Controller1/1 -> Sum1/1  "PI"
  Sum7/1 -> [eqref]
  Constant6/1 -> Product1/1
  [vd] -> Sum3/2, Gain9/1
  Gain10/1 -> Sum1/2
  PID Controller4/1 -> Sum13/2  "PI"
  [vqref] -> Sum4/2
  Gain2/1 -> Sum7/1
  Product/1 -> [kpv]
  Constant5/1 -> Product/1
  [id] -> Gain2/1, Sum5/2
  [vdref] -> Sum3/1
  [kpv] -> PID Controller1/2
  PID Controller2/1 -> Sum2/1  "PI"

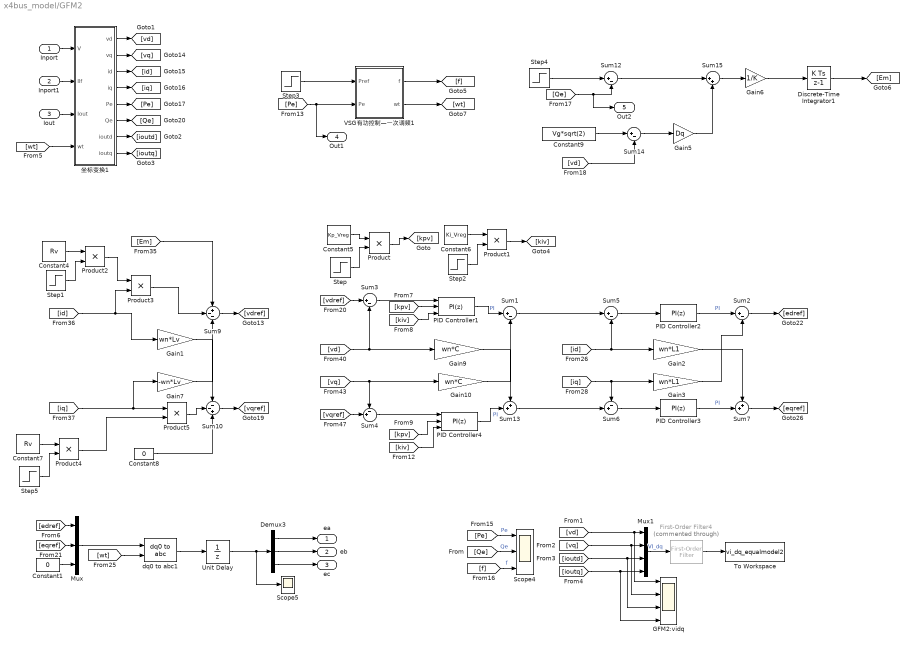
== system x4bus_model/GFM2 ==
  Inport : Inport
  Inport1 : Inport  Port=2
  Iout : Inport  Port=3
  Constant1 : Constant  Value=0
  Constant4 : Constant  Value=Rv
  Constant5 : Constant  Value=Kp_Vreg
  Constant6 : Constant  Value=Ki_Vreg
  Constant7 : Constant  Value=Rv
  Constant8 : Constant  Value=0
  Constant9 : Constant  Value=Vg*sqrt(2)
  Demux3 : Demux  Outputs=3
  Discrete-Time Integrator1 : DiscreteIntegrator  SampleTime=-1  ICPrevOutput=DiscIntNeverNeededParam  ICPrevScaledInput=DiscIntNeverNeededParam
  First-Order Filter4 : spsFirstOrderFilterLib/First-Order Filter  Commented=through  FilterType=Lowpass  Tc=5e-3  Ts=Ts  Initialize=off  Vac_Init=[0, 0, 1000]  Vdc_Init=0  PlotResponse=off  FreqRange="[0,  200,  1]"
  GFM2:vidq : Scope  NumInputPorts=4
  Gain1 : Gain  Gain=wn*Lv
  Gain10 : Gain  Gain=wn*C
  Gain2 : Gain  Gain=wn*L1
  Gain3 : Gain  Gain=wn*L1
  Gain5 : Gain  Gain=Dq
  Gain6 : Gain  Gain=1/K
  Gain7 : Gain  Gain=-wn*Lv
  Gain9 : Gain  Gain=wn*C
  Mux : Mux  Inputs=3
  Mux1 : Mux
  PID Controller1 : slpidlib/PID Controller  Controller=PI  Form=Parallel  TimeDomain=Discrete-time  UseExternalTs=off  SampleTime=-1  IntegratorMethod=Forward Euler  FilterMethod=Forward Euler  ControllerParametersSource=external  P=Kp_Vreg  I=Ki_Vreg  UseKiTs=off  D=0  UseExternalDerivativeSource=off  N=100  UseFilter=on  TunerSelectOption=Transfer Function Based (PID Tuner App)  InitialConditionSource=internal  InitialConditionForIntegrator=0  InitialConditionForFilter=0  DifferentiatorICPrevScaledInput=0  ExternalReset=none  TrackingMode=off  Kt=1  LimitOutput=off  SatLimitsSource=internal  UpperSaturationLimit=inf  LowerSaturationLimit=-inf  LinearizeAsGain=on  AntiWindupMode=none  Kb=1  LimitIntegrator=off  UpperIntegratorSaturationLimit=inf  LowerIntegratorSaturationLimit=-inf  POutMin=[]  POutMax=[]  IOutMin=[]  IOutMax=[]  DOutMin=[]  DOutMax=[]  NOutMin=[]  NOutMax=[]  SumOutMin=[]  SumOutMax=[]  SaturationOutMin=[]  SaturationOutMax=[]  PParamMin=[]  PParamMax=[]  IParamMin=[]  IParamMax=[]  DParamMin=[]  DParamMax=[]  NParamMin=[]  NParamMax=[]  KbParamMin=[]  KbParamMax=[]  KtParamMin=[]  KtParamMax=[]  KbOutMin=[]  KbOutMax=[]  KtOutMin=[]  KtOutMax=[]  IntegratorOutMin=[]  IntegratorOutMax=[]  FilterOutMin=[]  FilterOutMax=[]  SumI1OutMin=[]  SumI1OutMax=[]  SumI2OutMin=[]  SumI2OutMax=[]  SumI3OutMin=[]  SumI3OutMax=[]  SumI4OutMin=[]  SumI4OutMax=[]  SumDOutMin=[]  SumDOutMax=[]  DifferentiatorOutMin=[]  DifferentiatorOutMax=[]  FilterDiffOutCoefMin=[]  FilterDiffOutCoefMax=[]  ReciprocalOutMin=[]  ReciprocalOutMax=[]  SumDenOutMin=[]  SumDenOutMax=[]  SumNumOutMin=[]  SumNumOutMax=[]  DivideOutMin=[]  DivideOutMax=[]  UdiffTsProdOutMin=[]  UdiffTsProdOutMax=[]  NTsProdOutMin=[]  NTsProdOutMax=[]  UintegralTsProdOutMin=[]  UintegralTsProdOutMax=[]  UngainTsProdOutMin=[]  UngainTsProdOutMax=[]  ClampingZeroOutDataTypeStr=Inherit: Inherit via back propagation  ClampingZeroOutMin=[]  ClampingZeroOutMax=[]  FilterDenConstantOutDataTypeStr=Inherit: Inherit via back propagation  FilterDenConstantOutMin=[]  FilterDenConstantOutMax=[]  PCopyOutDataTypeStr=Inherit: Inherit via back propagation  PCopyOutMin=[]  PCopyOutMax=[]  NCopyOutDataTypeStr=Inherit: Inherit via back propagation  NCopyOutMin=[]  NCopyOutMax=[]  IntegratorContinuousStateAttributes=''  IntegratorStateMustResolveToSignalObject=off  IntegratorRTWStateStorageClass=Auto  FilterContinuousStateAttributes=''  FilterStateMustResolveToSignalObject=off  FilterRTWStateStorageClass=Auto  ParallelPVariant=ExternalParameters  IdealPVariant=Disabled  IVariant=ExternalParameters  DVariant=Disabled  IntegratorVariant=Discrete  SatVariant=Disabled  AWVariant=Passthrough  PCopyVariant=Disabled  TRVariant=Disabled  FdbkBlocksVariant=Forward  IdealPFdbkVariant=Disabled  SatFdbkVariant=Disabled  DerivativeFilterVariant=Disabled  NVariant=Disabled  NCopyVariant=Disabled_SignalSpec  FilterICVariant=Disabled  IntegratorICVariant=InternalICs  ExternalResetVariant=Disabled  TRSumVariant=Passthrough  SumFdbkVariant=Disabled  SumVariant=Sum_PI  TsampFilterVariant=InternalTs  TsampNgainVariant=Passthrough  TsampIntegralVariant=Disabled_SignalSpec  ExternalSaturationOutDataTypeStr=Inherit: Same as second input  DerivativeSourceVariant=Disabled  PreIntVariant=InternalPreInt
  PID Controller2 : slpidlib/PID Controller  Controller=PI  Form=Parallel  TimeDomain=Discrete-time  UseExternalTs=off  SampleTime=-1  IntegratorMethod=Forward Euler  FilterMethod=Forward Euler  ControllerParametersSource=internal  P=Kp_Ireg  I=Ki_Ireg  UseKiTs=off  D=0  UseExternalDerivativeSource=off  N=100  UseFilter=on  TunerSelectOption=Transfer Function Based (PID Tuner App)  InitialConditionSource=internal  InitialConditionForIntegrator=0  InitialConditionForFilter=0  DifferentiatorICPrevScaledInput=0  ExternalReset=none  TrackingMode=off  Kt=1  LimitOutput=off  SatLimitsSource=internal  UpperSaturationLimit=inf  LowerSaturationLimit=-inf  LinearizeAsGain=on  AntiWindupMode=none  Kb=1  LimitIntegrator=off  UpperIntegratorSaturationLimit=inf  LowerIntegratorSaturationLimit=-inf  POutMin=[]  POutMax=[]  IOutMin=[]  IOutMax=[]  DOutMin=[]  DOutMax=[]  NOutMin=[]  NOutMax=[]  SumOutMin=[]  SumOutMax=[]  SaturationOutMin=[]  SaturationOutMax=[]  PParamMin=[]  PParamMax=[]  IParamMin=[]  IParamMax=[]  DParamMin=[]  DParamMax=[]  NParamMin=[]  NParamMax=[]  KbParamMin=[]  KbParamMax=[]  KtParamMin=[]  KtParamMax=[]  KbOutMin=[]  KbOutMax=[]  KtOutMin=[]  KtOutMax=[]  IntegratorOutMin=[]  IntegratorOutMax=[]  FilterOutMin=[]  FilterOutMax=[]  SumI1OutMin=[]  SumI1OutMax=[]  SumI2OutMin=[]  SumI2OutMax=[]  SumI3OutMin=[]  SumI3OutMax=[]  SumI4OutMin=[]  SumI4OutMax=[]  SumDOutMin=[]  SumDOutMax=[]  DifferentiatorOutMin=[]  DifferentiatorOutMax=[]  FilterDiffOutCoefMin=[]  FilterDiffOutCoefMax=[]  ReciprocalOutMin=[]  ReciprocalOutMax=[]  SumDenOutMin=[]  SumDenOutMax=[]  SumNumOutMin=[]  SumNumOutMax=[]  DivideOutMin=[]  DivideOutMax=[]  UdiffTsProdOutMin=[]  UdiffTsProdOutMax=[]  NTsProdOutMin=[]  NTsProdOutMax=[]  UintegralTsProdOutMin=[]  UintegralTsProdOutMax=[]  UngainTsProdOutMin=[]  UngainTsProdOutMax=[]  ClampingZeroOutDataTypeStr=Inherit: Inherit via back propagation  ClampingZeroOutMin=[]  ClampingZeroOutMax=[]  FilterDenConstantOutDataTypeStr=Inherit: Inherit via back propagation  FilterDenConstantOutMin=[]  FilterDenConstantOutMax=[]  PCopyOutDataTypeStr=Inherit: Inherit via back propagation  PCopyOutMin=[]  PCopyOutMax=[]  NCopyOutDataTypeStr=Inherit: Inherit via back propagation  NCopyOutMin=[]  NCopyOutMax=[]  IntegratorContinuousStateAttributes=''  IntegratorStateMustResolveToSignalObject=off  IntegratorRTWStateStorageClass=Auto  FilterContinuousStateAttributes=''  FilterStateMustResolveToSignalObject=off  FilterRTWStateStorageClass=Auto  ParallelPVariant=InternalParameters  IdealPVariant=Disabled  IVariant=InternalParameters  DVariant=Disabled  IntegratorVariant=Discrete  SatVariant=Disabled  AWVariant=Passthrough  PCopyVariant=Disabled  TRVariant=Disabled  FdbkBlocksVariant=Forward  IdealPFdbkVariant=Disabled  SatFdbkVariant=Disabled  DerivativeFilterVariant=Disabled  NVariant=Disabled  NCopyVariant=Disabled_SignalSpec  FilterICVariant=Disabled  IntegratorICVariant=InternalICs  ExternalResetVariant=Disabled  TRSumVariant=Passthrough  SumFdbkVariant=Disabled  SumVariant=Sum_PI  TsampFilterVariant=InternalTs  TsampNgainVariant=Passthrough  TsampIntegralVariant=Disabled_SignalSpec  ExternalSaturationOutDataTypeStr=Inherit: Same as second input  DerivativeSourceVariant=Disabled  PreIntVariant=InternalPreInt
  PID Controller3 : slpidlib/PID Controller  Controller=PI  Form=Parallel  TimeDomain=Discrete-time  UseExternalTs=off  SampleTime=-1  IntegratorMethod=Forward Euler  FilterMethod=Forward Euler  ControllerParametersSource=internal  P=Kp_Ireg  I=Ki_Ireg  UseKiTs=off  D=0  UseExternalDerivativeSource=off  N=100  UseFilter=on  TunerSelectOption=Transfer Function Based (PID Tuner App)  InitialConditionSource=internal  InitialConditionForIntegrator=0  InitialConditionForFilter=0  DifferentiatorICPrevScaledInput=0  ExternalReset=none  TrackingMode=off  Kt=1  LimitOutput=off  SatLimitsSource=internal  UpperSaturationLimit=inf  LowerSaturationLimit=-inf  LinearizeAsGain=on  AntiWindupMode=none  Kb=1  LimitIntegrator=off  UpperIntegratorSaturationLimit=inf  LowerIntegratorSaturationLimit=-inf  POutMin=[]  POutMax=[]  IOutMin=[]  IOutMax=[]  DOutMin=[]  DOutMax=[]  NOutMin=[]  NOutMax=[]  SumOutMin=[]  SumOutMax=[]  SaturationOutMin=[]  SaturationOutMax=[]  PParamMin=[]  PParamMax=[]  IParamMin=[]  IParamMax=[]  DParamMin=[]  DParamMax=[]  NParamMin=[]  NParamMax=[]  KbParamMin=[]  KbParamMax=[]  KtParamMin=[]  KtParamMax=[]  KbOutMin=[]  KbOutMax=[]  KtOutMin=[]  KtOutMax=[]  IntegratorOutMin=[]  IntegratorOutMax=[]  FilterOutMin=[]  FilterOutMax=[]  SumI1OutMin=[]  SumI1OutMax=[]  SumI2OutMin=[]  SumI2OutMax=[]  SumI3OutMin=[]  SumI3OutMax=[]  SumI4OutMin=[]  SumI4OutMax=[]  SumDOutMin=[]  SumDOutMax=[]  DifferentiatorOutMin=[]  DifferentiatorOutMax=[]  FilterDiffOutCoefMin=[]  FilterDiffOutCoefMax=[]  ReciprocalOutMin=[]  ReciprocalOutMax=[]  SumDenOutMin=[]  SumDenOutMax=[]  SumNumOutMin=[]  SumNumOutMax=[]  DivideOutMin=[]  DivideOutMax=[]  UdiffTsProdOutMin=[]  UdiffTsProdOutMax=[]  NTsProdOutMin=[]  NTsProdOutMax=[]  UintegralTsProdOutMin=[]  UintegralTsProdOutMax=[]  UngainTsProdOutMin=[]  UngainTsProdOutMax=[]  ClampingZeroOutDataTypeStr=Inherit: Inherit via back propagation  ClampingZeroOutMin=[]  ClampingZeroOutMax=[]  FilterDenConstantOutDataTypeStr=Inherit: Inherit via back propagation  FilterDenConstantOutMin=[]  FilterDenConstantOutMax=[]  PCopyOutDataTypeStr=Inherit: Inherit via back propagation  PCopyOutMin=[]  PCopyOutMax=[]  NCopyOutDataTypeStr=Inherit: Inherit via back propagation  NCopyOutMin=[]  NCopyOutMax=[]  IntegratorContinuousStateAttributes=''  IntegratorStateMustResolveToSignalObject=off  IntegratorRTWStateStorageClass=Auto  FilterContinuousStateAttributes=''  FilterStateMustResolveToSignalObject=off  FilterRTWStateStorageClass=Auto  ParallelPVariant=InternalParameters  IdealPVariant=Disabled  IVariant=InternalParameters  DVariant=Disabled  IntegratorVariant=Discrete  SatVariant=Disabled  AWVariant=Passthrough  PCopyVariant=Disabled  TRVariant=Disabled  FdbkBlocksVariant=Forward  IdealPFdbkVariant=Disabled  SatFdbkVariant=Disabled  DerivativeFilterVariant=Disabled  NVariant=Disabled  NCopyVariant=Disabled_SignalSpec  FilterICVariant=Disabled  IntegratorICVariant=InternalICs  ExternalResetVariant=Disabled  TRSumVariant=Passthrough  SumFdbkVariant=Disabled  SumVariant=Sum_PI  TsampFilterVariant=InternalTs  TsampNgainVariant=Passthrough  TsampIntegralVariant=Disabled_SignalSpec  ExternalSaturationOutDataTypeStr=Inherit: Same as second input  DerivativeSourceVariant=Disabled  PreIntVariant=InternalPreInt
  PID Controller4 : slpidlib/PID Controller  Controller=PI  Form=Parallel  TimeDomain=Discrete-time  UseExternalTs=off  SampleTime=-1  IntegratorMethod=Forward Euler  FilterMethod=Forward Euler  ControllerParametersSource=external  P=Kp_Vreg  I=Ki_Vreg  UseKiTs=off  D=0  UseExternalDerivativeSource=off  N=100  UseFilter=on  TunerSelectOption=Transfer Function Based (PID Tuner App)  InitialConditionSource=internal  InitialConditionForIntegrator=0  InitialConditionForFilter=0  DifferentiatorICPrevScaledInput=0  ExternalReset=none  TrackingMode=off  Kt=1  LimitOutput=off  SatLimitsSource=internal  UpperSaturationLimit=inf  LowerSaturationLimit=-inf  LinearizeAsGain=on  AntiWindupMode=none  Kb=1  LimitIntegrator=off  UpperIntegratorSaturationLimit=inf  LowerIntegratorSaturationLimit=-inf  POutMin=[]  POutMax=[]  IOutMin=[]  IOutMax=[]  DOutMin=[]  DOutMax=[]  NOutMin=[]  NOutMax=[]  SumOutMin=[]  SumOutMax=[]  SaturationOutMin=[]  SaturationOutMax=[]  PParamMin=[]  PParamMax=[]  IParamMin=[]  IParamMax=[]  DParamMin=[]  DParamMax=[]  NParamMin=[]  NParamMax=[]  KbParamMin=[]  KbParamMax=[]  KtParamMin=[]  KtParamMax=[]  KbOutMin=[]  KbOutMax=[]  KtOutMin=[]  KtOutMax=[]  IntegratorOutMin=[]  IntegratorOutMax=[]  FilterOutMin=[]  FilterOutMax=[]  SumI1OutMin=[]  SumI1OutMax=[]  SumI2OutMin=[]  SumI2OutMax=[]  SumI3OutMin=[]  SumI3OutMax=[]  SumI4OutMin=[]  SumI4OutMax=[]  SumDOutMin=[]  SumDOutMax=[]  DifferentiatorOutMin=[]  DifferentiatorOutMax=[]  FilterDiffOutCoefMin=[]  FilterDiffOutCoefMax=[]  ReciprocalOutMin=[]  ReciprocalOutMax=[]  SumDenOutMin=[]  SumDenOutMax=[]  SumNumOutMin=[]  SumNumOutMax=[]  DivideOutMin=[]  DivideOutMax=[]  UdiffTsProdOutMin=[]  UdiffTsProdOutMax=[]  NTsProdOutMin=[]  NTsProdOutMax=[]  UintegralTsProdOutMin=[]  UintegralTsProdOutMax=[]  UngainTsProdOutMin=[]  UngainTsProdOutMax=[]  ClampingZeroOutDataTypeStr=Inherit: Inherit via back propagation  ClampingZeroOutMin=[]  ClampingZeroOutMax=[]  FilterDenConstantOutDataTypeStr=Inherit: Inherit via back propagation  FilterDenConstantOutMin=[]  FilterDenConstantOutMax=[]  PCopyOutDataTypeStr=Inherit: Inherit via back propagation  PCopyOutMin=[]  PCopyOutMax=[]  NCopyOutDataTypeStr=Inherit: Inherit via back propagation  NCopyOutMin=[]  NCopyOutMax=[]  IntegratorContinuousStateAttributes=''  IntegratorStateMustResolveToSignalObject=off  IntegratorRTWStateStorageClass=Auto  FilterContinuousStateAttributes=''  FilterStateMustResolveToSignalObject=off  FilterRTWStateStorageClass=Auto  ParallelPVariant=ExternalParameters  IdealPVariant=Disabled  IVariant=ExternalParameters  DVariant=Disabled  IntegratorVariant=Discrete  SatVariant=Disabled  AWVariant=Passthrough  PCopyVariant=Disabled  TRVariant=Disabled  FdbkBlocksVariant=Forward  IdealPFdbkVariant=Disabled  SatFdbkVariant=Disabled  DerivativeFilterVariant=Disabled  NVariant=Disabled  NCopyVariant=Disabled_SignalSpec  FilterICVariant=Disabled  IntegratorICVariant=InternalICs  ExternalResetVariant=Disabled  TRSumVariant=Passthrough  SumFdbkVariant=Disabled  SumVariant=Sum_PI  TsampFilterVariant=InternalTs  TsampNgainVariant=Passthrough  TsampIntegralVariant=Disabled_SignalSpec  ExternalSaturationOutDataTypeStr=Inherit: Same as second input  DerivativeSourceVariant=Disabled  PreIntVariant=InternalPreInt
  Product{,1..5} (6 alike) : Product
  Scope4 : Scope  NumInputPorts=3
  Scope5 : Scope
  Step : Step  Time=t2  Before=1  After=0.85  SampleTime=0
  Step1 : Step  Time=t2  Before=1  SampleTime=0
  Step2 : Step  Time=t2  Before=1  After=0.9  SampleTime=0
  Step3 : Step  Time=t2  Before=Po  After=0.8*Po  SampleTime=0
  Step4 : Step  Time=t2  Before=Qo  After=0.1*Po  SampleTime=0
  Step5 : Step  Time=t2  Before=1  SampleTime=0
  Sum{1..3,5,12,14} (6 alike) : Sum  Inputs=|+-
  Sum10 : Sum  Inputs=--+
  Sum13 : Sum  Inputs=++|
  Sum15 : Sum  Inputs=|++
  Sum4 : Sum  Inputs=-+|
  Sum6 : Sum  Inputs=-+|
  Sum7 : Sum  Inputs=++|
  Sum9 : Sum  Inputs=+--
  To Workspace : ToWorkspace  VariableName=vi_dq_equalmodel2  SaveFormat=Timeseries  SampleTime=-1
  Unit Delay : UnitDelay  SampleTime=-1  HasFrameUpgradeWarning=on
  VSG有功控制—一次调频1 : Subsystem
  dq0 to abc1 : spsdq0toabcLib/dq0 to abc  Alignment=90 degrees behind phase A axis
  坐标变换1 : Subsystem
  ea : Outport
  eb : Outport  Port=2
  ec : Outport  Port=3
  Out1 : Outport  Port=4
  Out2 : Outport  Port=5
  wires:
  Iout/1 -> 坐标变换1/3(Iout)
  坐标变换1/7(ioutd) -> [ioutd]
  坐标变换1/8(ioutq) -> [ioutq]
  Inport/1 -> 坐标变换1/1(V)
  Unit Delay/1 -> Demux3/1, Scope5/1
  Demux3/3 -> ec/1
  Demux3/2 -> eb/1
  Demux3/1 -> ea/1
  dq0 to abc1/1 -> Unit Delay/1
  Constant1/1 -> Mux/3
  Mux/1 -> dq0 to abc1/1
  [eqref] -> Mux/2
  [edref] -> Mux/1
  [wt] -> dq0 to abc1/2
  坐标变换1/6(Qe) -> [Qe]
  坐标变换1/5(Pe) -> [Pe]
  坐标变换1/4(iq) -> [iq]
  坐标变换1/3(id) -> [id]
  坐标变换1/2(vq) -> [vq]
  坐标变换1/1(vd) -> [vd]
  [wt] -> 坐标变换1/4(wt)
  Inport1/1 -> 坐标变换1/2(Ilf)
  First-Order Filter4/1 -> To Workspace/1
  Mux1/1 -> First-Order Filter4/1  "VI_dq"
  [ioutq] -> Mux1/4, GFM2:vidq/4
  [vd] -> Mux1/1, GFM2:vidq/1
  [ioutd] -> Mux1/3, GFM2:vidq/3
  [vq] -> Mux1/2, GFM2:vidq/2
  [Qe] -> Scope4/2  "Qe"
  [f] -> Scope4/3  "f"
  [Pe] -> Scope4/1  "Pe"
  Step1/1 -> Product2/2
  Product/1 -> [kpv]
  Step2/1 -> Product1/2
  Product5/1 -> Sum10/2
  Product4/1 -> Product5/2
  Step5/1 -> Product4/2
  Product1/1 -> [kiv]
  [kpv] -> PID Controller1/2
  PID Controller4/1 -> Sum13/2  "PI"
  Constant5/1 -> Product/1
  Gain3/1 -> Sum2/2
  [iq] -> Gain7/1, Product5/1
  [iq] -> Sum6/1, Gain3/1
  Sum9/1 -> [vdref]
  Sum10/1 -> [vqref]
  Sum7/1 -> [eqref]
  [Em] -> Sum9/1
  Constant8/1 -> Sum10/3
  Sum3/1 -> PID Controller1/1
  [vqref] -> Sum4/2
  [vq] -> Gain10/1, Sum4/1
  Constant4/1 -> Product2/1
  PID Controller2/1 -> Sum2/1  "PI"
  Constant7/1 -> Product4/1
  [id] -> Gain2/1, Sum5/2
  Sum5/1 -> PID Controller2/1
  [vdref] -> Sum3/1
  Gain1/1 -> Sum10/1
  Product3/1 -> Sum9/2
  Gain2/1 -> Sum7/1
  Gain7/1 -> Sum9/3
  Sum2/1 -> [edref]
  PID Controller1/1 -> Sum1/1  "PI"
  Sum6/1 -> PID Controller3/1
  [kpv] -> PID Controller4/2
  Sum4/1 -> PID Controller4/1
  [kiv] -> PID Controller4/3
  Sum1/1 -> Sum5/1
  Gain10/1 -> Sum1/2
  [vd] -> Sum3/2, Gain9/1
  [kiv] -> PID Controller1/3
  PID Controller3/1 -> Sum7/2  "PI"
  Step/1 -> Product/2
  Constant6/1 -> Product1/1
  Product2/1 -> Product3/1
  Sum13/1 -> Sum6/2
  Gain9/1 -> Sum13/1
  [id] -> Gain1/1, Product3/2
  Step4/1 -> Sum12/1
  VSG有功控制—一次调频1/2(wt) -> [wt]
  Sum12/1 -> Sum15/1
  [Pe] -> Out1/1, VSG有功控制—一次调频1/2(Pe)
  Sum14/1 -> Gain5/1
  Constant9/1 -> Sum14/1
  Sum15/1 -> Gain6/1
  [vd] -> Sum14/2
  VSG有功控制—一次调频1/1(f) -> [f]
  Gain6/1 -> Discrete-Time Integrator1/1
  Discrete-Time Integrator1/1 -> [Em]
  [Qe] -> Out2/1, Sum12/2
  Step3/1 -> VSG有功控制—一次调频1/1(Pref)
  Gain5/1 -> Sum15/2

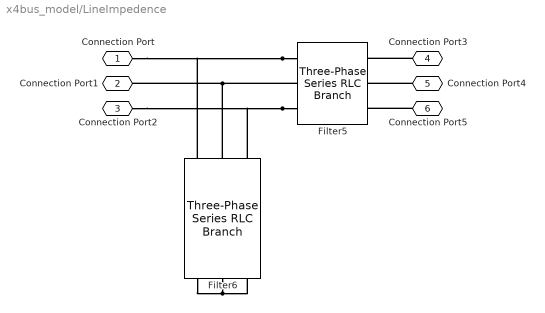
== system x4bus_model/LineImpedence ==
  Filter5 : spsThreePhaseSeriesRLCBranchLib/Three-Phase Series RLC Branch  LConnTagsString=A|B|C  RConnTagsString=A|B|C  BranchType=RL  Resistance=0.02904  Inductance=0.924e-3  Capacitance=1e-6  Measurements=None
  Filter6 : spsThreePhaseSeriesRLCBranchLib/Three-Phase Series RLC Branch  LConnTagsString=A|B|C  RConnTagsString=A|B|C  BranchType=RC  Resistance=0.001  Inductance=L2  Capacitance=657.6e-6  Measurements=None
  Connection Port : PMIOPort  Side=Left
  Connection Port1 : PMIOPort  Port=2  Side=Left
  Connection Port2 : PMIOPort  Port=3  Side=Left
  Connection Port3 : PMIOPort  Port=4  Side=Right
  Connection Port4 : PMIOPort  Port=5  Side=Right
  Connection Port5 : PMIOPort  Port=6  Side=Right
  connections:
  Connection Port5/RConn1 -- Filter5/RConn3
  Filter5/LConn3 -- Connection Port2/RConn1 -- Filter6/LConn3
  Filter6/RConn1 -- Filter6/RConn2 -- Filter6/RConn3
  Filter5/LConn1 -- Connection Port/RConn1 -- Filter6/LConn1
  Connection Port4/RConn1 -- Filter5/RConn2
  Filter5/LConn2 -- Connection Port1/RConn1 -- Filter6/LConn2
  Connection Port3/RConn1 -- Filter5/RConn1

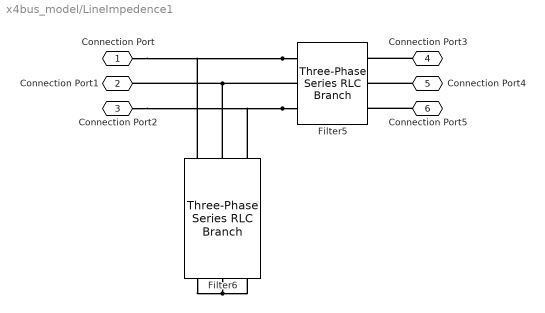
== system x4bus_model/LineImpedence1 ==
  Filter5 : spsThreePhaseSeriesRLCBranchLib/Three-Phase Series RLC Branch  LConnTagsString=A|B|C  RConnTagsString=A|B|C  BranchType=RL  Resistance=0.02904  Inductance=0.924e-3  Capacitance=1e-6  Measurements=None
  Filter6 : spsThreePhaseSeriesRLCBranchLib/Three-Phase Series RLC Branch  LConnTagsString=A|B|C  RConnTagsString=A|B|C  BranchType=RC  Resistance=0.001  Inductance=L2  Capacitance=657.6e-6  Measurements=None
  Connection Port : PMIOPort  Side=Left
  Connection Port1 : PMIOPort  Port=2  Side=Left
  Connection Port2 : PMIOPort  Port=3  Side=Left
  Connection Port3 : PMIOPort  Port=4  Side=Right
  Connection Port4 : PMIOPort  Port=5  Side=Right
  Connection Port5 : PMIOPort  Port=6  Side=Right
  connections:
  Filter5/LConn3 -- Connection Port2/RConn1 -- Filter6/LConn3
  Filter5/LConn2 -- Connection Port1/RConn1 -- Filter6/LConn2
  Filter5/LConn1 -- Connection Port/RConn1 -- Filter6/LConn1
  Filter6/RConn1 -- Filter6/RConn2 -- Filter6/RConn3
  Connection Port4/RConn1 -- Filter5/RConn2
  Connection Port5/RConn1 -- Filter5/RConn3
  Connection Port3/RConn1 -- Filter5/RConn1
